simulink model "EDDA_2nd"  (R2020a)
settings: Solver=ode45  StartTime=0.0  StopTime=T  RelTol=1e-6
values from neighbouring files (symbols this model uses):
  g = 9.81    [TestingIkRTR.m]    (also in TestingScript.m; TestingScriptRTR.m)
  Kd1 = Kp1/10    (= 100)    [TestingIkRTR.m]    (also in TestingScript.m; TestingScriptRTR.m)
  Kp1 = 1000    [TestingIkRTR.m]    (also in TestingScript.m; TestingScriptRTR.m)
  O1 = 3.1    [TestingScript.m]
  O2 = 9.5    [TestingScript.m]
  O3 = 0.24    [TestingScript.m]
  O4 = 0.77    [TestingScript.m]
settings Model: Creator=ja  LastModifiedBy=ja

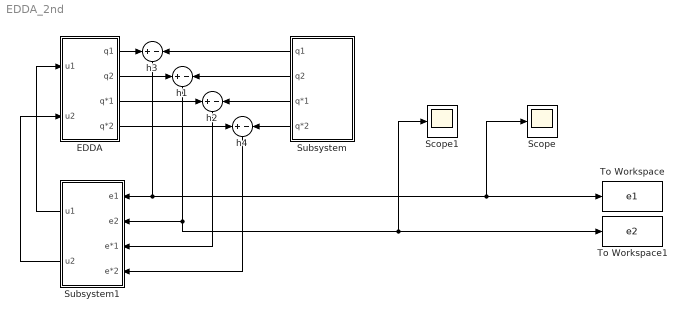
== system EDDA_2nd ==
  EDDA : Subsystem
  Scope : Scope
  Scope1 : Scope
  Subsystem : Subsystem
  Subsystem1 : Subsystem
  To Workspace : ToWorkspace  VariableName=e1  SampleTime=-1
  To Workspace1 : ToWorkspace  VariableName=e2  SampleTime=-1
  h{1..4} (4 alike) : Sum  Inputs=+-
  wires:
  EDDA/1(q1) -> h3/1
  Subsystem/1(q1) -> h3/2
  EDDA/2(q2) -> h1/1
  Subsystem/2(q2) -> h1/2
  EDDA/3(q*1) -> h2/1
  Subsystem/3(q*1) -> h2/2
  Subsystem/4(q*2) -> h4/2
  EDDA/4(q*2) -> h4/1
  h3/1 -> Subsystem1/1(e1), Scope/1, To Workspace/1
  h1/1 -> Scope1/1, To Workspace1/1, Subsystem1/2(e2)
  h2/1 -> Subsystem1/3(e*1)
  h4/1 -> Subsystem1/4(e*2)
  Subsystem1/1(u1) -> EDDA/1(u1)
  Subsystem1/2(u2) -> EDDA/2(u2)

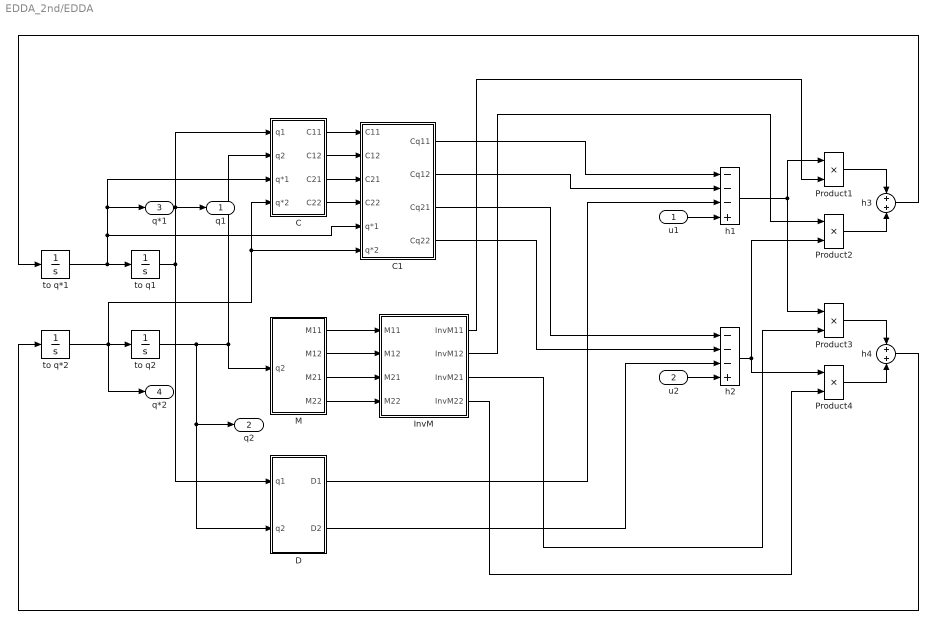
== system EDDA_2nd/EDDA ==
  u1 : Inport
  u2 : Inport  Port=2
  C : Subsystem
  C1 : Subsystem
  D : Subsystem
  InvM : MATLAB Function  TreatAsAtomicUnit=on
  M : Subsystem
  Product{1..4} (4 alike) : Product
  h1 : Sum  Inputs=---+
  h2 : Sum  Inputs=---+
  h3 : Sum
  h4 : Sum
  to q*1 : Integrator
  to q*2 : Integrator
  to q1 : Integrator
  to q2 : Integrator
  q1 : Outport
  q2 : Outport  Port=2
  q*1 : Outport  Port=3
  q*2 : Outport  Port=4
  wires:
  C/4(C22) -> C1/4(C22)
  to q*2/1 -> q*2/1, C1/6(q*2), C/4(q*2), to q2/1
  C/3(C21) -> C1/3(C21)
  u1/1 -> h1/4
  InvM/3(InvM21) -> Product3/2
  u2/1 -> h2/4
  to q*1/1 -> q*1/1, C/3(q*1), C1/5(q*1), to q1/1
  Product3/1 -> h4/1
  C/2(C12) -> C1/2(C12)
  C1/1(Cq11) -> h1/1
  h1/1 -> Product1/1, Product3/1
  to q1/1 -> D/1(q1), q1/1, C/1(q1)
  h2/1 -> Product4/1, Product2/2
  to q2/1 -> C/2(q2), M/1(q2), q2/1, D/2(q2)
  InvM/4(InvM22) -> Product4/2
  M/1(M11) -> InvM/1(M11)
  h3/1 -> to q*1/1
  M/3(M21) -> InvM/3(M21)
  M/2(M12) -> InvM/2(M12)
  M/4(M22) -> InvM/4(M22)
  D/1(D1) -> h1/3
  C/1(C11) -> C1/1(C11)
  InvM/2(InvM12) -> Product2/1
  Product1/1 -> h3/1
  C1/4(Cq22) -> h2/2
  C1/3(Cq21) -> h2/1
  Product4/1 -> h4/2
  C1/2(Cq12) -> h1/2
  InvM/1(InvM11) -> Product1/2
  D/2(D2) -> h2/3
  h4/1 -> to q*2/1
  Product2/1 -> h3/2

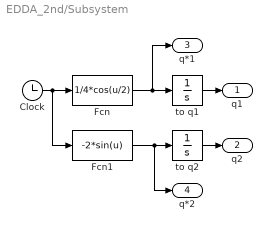
== system EDDA_2nd/Subsystem ==
  Clock : Clock
  Fcn : Fcn  Expr=1/4*cos(u/2)
  Fcn1 : Fcn  Expr=-2*sin(u)
  to q1 : Integrator
  to q2 : Integrator  InitialCondition=2
  q1 : Outport
  q2 : Outport  Port=2
  q*1 : Outport  Port=3
  q*2 : Outport  Port=4
  wires:
  Fcn1/1 -> q*2/1, to q2/1
  to q2/1 -> q2/1
  Clock/1 -> Fcn1/1, Fcn/1
  to q1/1 -> q1/1
  Fcn/1 -> q*1/1, to q1/1

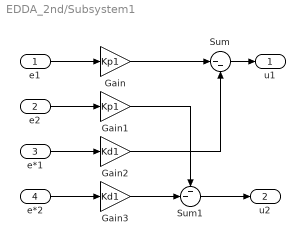
== system EDDA_2nd/Subsystem1 ==
  e1 : Inport
  e2 : Inport  Port=2
  e*1 : Inport  Port=3
  e*2 : Inport  Port=4
  Gain : Gain  Gain=Kp1
  Gain1 : Gain  Gain=Kp1
  Gain2 : Gain  Gain=Kd1
  Gain3 : Gain  Gain=Kd1
  Sum : Sum  Inputs=|--
  Sum1 : Sum  Inputs=--|
  u1 : Outport
  u2 : Outport  Port=2
  wires:
  e2/1 -> Gain1/1
  e1/1 -> Gain/1
  e*1/1 -> Gain2/1
  e*2/1 -> Gain3/1
  Gain1/1 -> Sum1/1
  Gain3/1 -> Sum1/2
  Gain/1 -> Sum/1
  Gain2/1 -> Sum/2
  Sum/1 -> u1/1
  Sum1/1 -> u2/1

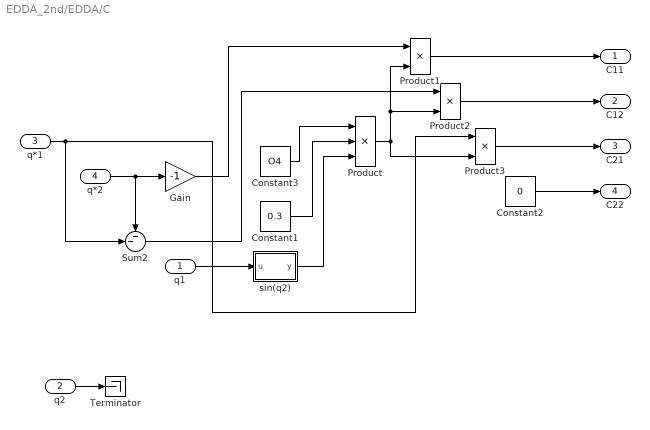
== system EDDA_2nd/EDDA/C ==
  q1 : Inport
  q2 : Inport  Port=2
  q*1 : Inport  Port=3
  q*2 : Inport  Port=4
  Constant1 : Constant  Value=0.3
  Constant2 : Constant  Value=0
  Constant3 : Constant  Value=O4
  Gain : Gain  Gain=-1
  Product : Product  Inputs=3
  Product1 : Product
  Product2 : Product
  Product3 : Product
  Sum2 : Sum  Inputs=--|
  Terminator : Terminator
  sin(q2) : MATLAB Function  TreatAsAtomicUnit=on
  C11 : Outport
  C12 : Outport  Port=2
  C21 : Outport  Port=3
  C22 : Outport  Port=4
  wires:
  q*2/1 -> Sum2/1, Gain/1
  sin(q2)/1(y) -> Product/3
  Constant1/1 -> Product/2
  Constant3/1 -> Product/1
  q2/1 -> Terminator/1
  Constant2/1 -> C22/1
  Product3/1 -> C21/1
  Product2/1 -> C12/1
  Product1/1 -> C11/1
  Product/1 -> Product1/2, Product2/2, Product3/2
  Gain/1 -> Product1/1
  q*1/1 -> Product3/1, Sum2/2
  Sum2/1 -> Product2/1
  q1/1 -> sin(q2)/1(u)

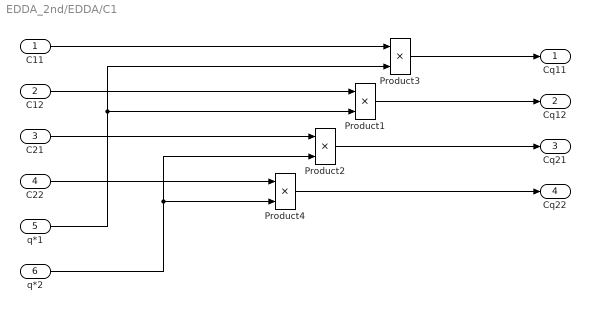
== system EDDA_2nd/EDDA/C1 ==
  C11 : Inport
  C12 : Inport  Port=2
  C21 : Inport  Port=3
  C22 : Inport  Port=4
  q*1 : Inport  Port=5
  q*2 : Inport  Port=6
  Product{1..4} (4 alike) : Product
  Cq11 : Outport
  Cq12 : Outport  Port=2
  Cq21 : Outport  Port=3
  Cq22 : Outport  Port=4
  wires:
  Product3/1 -> Cq11/1
  Product1/1 -> Cq12/1
  Product2/1 -> Cq21/1
  Product4/1 -> Cq22/1
  C22/1 -> Product4/1
  C21/1 -> Product2/1
  C12/1 -> Product1/1
  C11/1 -> Product3/1
  q*2/1 -> Product2/2, Product4/2
  q*1/1 -> Product3/2, Product1/2

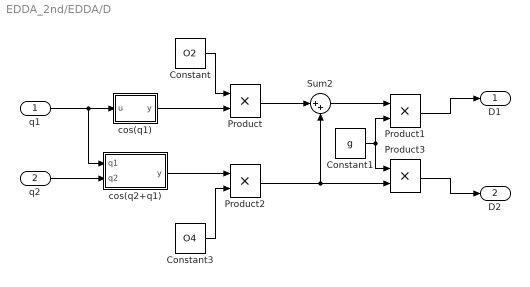
== system EDDA_2nd/EDDA/D ==
  q1 : Inport
  q2 : Inport  Port=2
  Constant : Constant  Value=O2
  Constant1 : Constant  Value=g
  Constant3 : Constant  Value=O4
  Product{,1..3} (4 alike) : Product
  Sum2 : Sum  Inputs=|++
  cos(q1) : MATLAB Function  TreatAsAtomicUnit=on
  cos(q2+q1) : MATLAB Function  TreatAsAtomicUnit=on
  D1 : Outport
  D2 : Outport  Port=2
  wires:
  cos(q1)/1(y) -> Product/2
  q1/1 -> cos(q2+q1)/1(q1), cos(q1)/1(u)
  q2/1 -> cos(q2+q1)/2(q2)
  cos(q2+q1)/1(y) -> Product2/1
  Product/1 -> Sum2/1
  Product2/1 -> Product3/2, Sum2/2
  Product3/1 -> D2/1
  Product1/1 -> D1/1
  Constant/1 -> Product/1
  Constant3/1 -> Product2/2
  Sum2/1 -> Product1/1
  Constant1/1 -> Product3/1, Product1/2

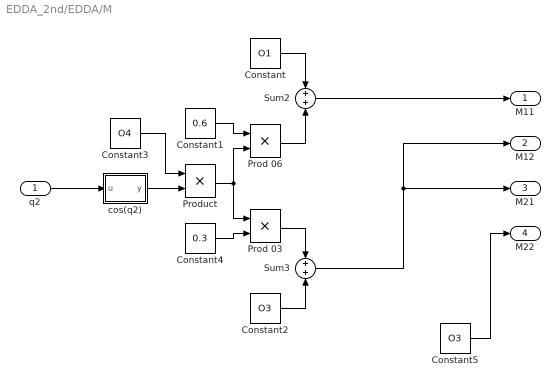
== system EDDA_2nd/EDDA/M ==
  q2 : Inport
  Constant : Constant  Value=O1
  Constant1 : Constant  Value=0.6
  Constant2 : Constant  Value=O3
  Constant3 : Constant  Value=O4
  Constant4 : Constant  Value=0.3
  Constant5 : Constant  Value=O3
  Prod 03 : Product
  Prod 06 : Product
  Product : Product
  Sum2 : Sum
  Sum3 : Sum
  cos(q2) : MATLAB Function  TreatAsAtomicUnit=on
  M11 : Outport
  M12 : Outport  Port=2
  M21 : Outport  Port=3
  M22 : Outport  Port=4
  wires:
  Constant4/1 -> Prod 03/2
  Prod 03/1 -> Sum3/1
  Product/1 -> Prod 03/1, Prod 06/2
  cos(q2)/1(y) -> Product/2
  Constant/1 -> Sum2/1
  Constant2/1 -> Sum3/2
  Constant3/1 -> Product/1
  Constant1/1 -> Prod 06/1
  Prod 06/1 -> Sum2/2
  q2/1 -> cos(q2)/1(u)
  Constant5/1 -> M22/1
  Sum3/1 -> M12/1, M21/1
  Sum2/1 -> M11/1

== matlab function EDDA_2nd/EDDA/M/cos(q2) ==
  data: u input; y output
function y = fcn(u)

y = cos(u);

== matlab function EDDA_2nd/EDDA/InvM ==
  data: M11 input; InvM11 output; M12 input; M21 input; M22 input; InvM12 output; InvM21 output; InvM22 output
function [InvM11, InvM12, InvM21, InvM22] = fcn(M11, M12, M21, M22)

M = [M11 M12; M21 M22];
M = inv(M);

InvM11 = M(1);
InvM12 = M(2);
InvM21 = M(3);
InvM22 = M(4);

== matlab function EDDA_2nd/EDDA/C/sin(q2) ==
  data: u input; y output
function y = fcn(u)

y = sin(u);

== matlab function EDDA_2nd/EDDA/D/cos(q1) ==
  data: u input; y output
function y = fcn(u)

y = cos(u);

== matlab function EDDA_2nd/EDDA/D/cos(q2+q1) ==
  data: q1 input; y output; q2 input
function y  = fcn(q1, q2)

y = cos(q1 + q2);
